simulink model "ex3"  (R2020a)
settings: Solver=ode45  StartTime=0.0  StopTime=1000  MaxStep=1e-3  RelTol=1e-3
libraries: cstblocks x5, simulink x1
settings Model: Creator=EREN  LastModifiedBy=EREN

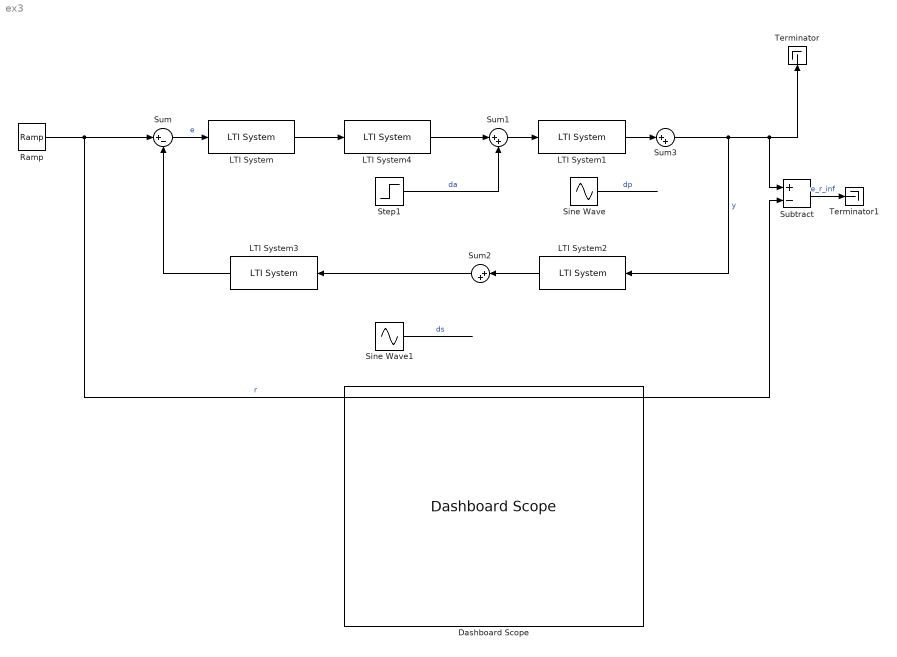
== system ex3 ==
  Dashboard Scope : DashboardScope
  LTI System : cstblocks/LTI System  sys=Gc  IC=[]
  LTI System1 : cstblocks/LTI System  sys=Gp  IC=[]
  LTI System2 : cstblocks/LTI System  sys=Gs  IC=[]
  LTI System3 : cstblocks/LTI System  sys=Gf  IC=[]
  LTI System4 : cstblocks/LTI System  sys=Ga  IC=[]
  Ramp : simulink/Sources/Ramp  slope=1  start=0  InitialOutput=0
  Sine Wave : Sin  Amplitude=16*10^-2  Frequency=0.03  SampleTime=0
  Sine Wave1 : Sin  Amplitude=2*10^-1  Frequency=60  SampleTime=0
  Step1 : Step  Time=0  After=1.5*10^-3  SampleTime=0
  Subtract : Sum  Inputs=+-
  Sum : Sum  Inputs=|+-
  Sum1 : Sum  Inputs=|++
  Sum2 : Sum  Inputs=|++
  Sum3 : Sum  Inputs=|++
  Terminator : Terminator
  Terminator1 : Terminator
  wires:
  Ramp/1 -> Subtract/2, Sum/1  "r"
  Sum/1 -> LTI System/1  "e"
  Sum1/1 -> LTI System1/1
  LTI System2/1 -> Sum2/1
  Sum2/1 -> LTI System3/1
  LTI System3/1 -> Sum/2
  LTI System1/1 -> Sum3/1
  Sum3/1 -> LTI System2/1, Subtract/1, Terminator/1  "y"
  Sine Wave1/1 -> ?  "ds"
  Sine Wave/1 -> ?  "dp"
  Step1/1 -> Sum1/2  "da"
  LTI System4/1 -> Sum1/1
  LTI System/1 -> LTI System4/1
  Subtract/1 -> Terminator1/1  "e_r_inf"
